simulink model "3_ZSM"  (R2016a)
settings: Solver=ode1  StartTime=0.0  StopTime=t_sim  FixedStep=0.001  RelTol=1e-3
values from neighbouring files (symbols this model uses):
  A = 1.5    [3_ZSM_Parameters.m]
  C = 1.3    [2_ESM_Parameters.m]    (also in 3_ZSM_Parameters.m)
  c_h_l = 0.5 * c_h    (= 71619.7243914)    [3_ZSM_Parameters.m]
  c_h_r = 0.5 * c_h    (= 71619.7243914)    [3_ZSM_Parameters.m]
  c_v_l = 0.5 * c_v    (= 39054.886799)    [3_ZSM_Parameters.m]
  c_v_r = 0.5 * c_v    (= 39054.886799)    [3_ZSM_Parameters.m]
  c_w = 0.4    [3_ZSM_Parameters.m]
  dynamicload_mode = i-1    [3_ZSM_Parameters.m]
  E = 0.85    [2_ESM_Parameters.m]    (also in 3_ZSM_Parameters.m)
  f_x_init = 0.5*A*c_w*rho*v_init^2    (= 24.980004)    [3_ZSM_Parameters.m]
  fz1 = fz(:,1)    [3_ZSM_Parameters.m]
  g = 9.81    [3_ZSM_Parameters.m]
  h_s = 0.5    [3_ZSM_Parameters.m]
  L = 2.71    [2_ESM_Parameters.m]    (also in 3_ZSM_Parameters.m)
  l_h = m_v * L / m    (= 1.35481930924)    [2_ESM_Parameters.m]    (also in 3_ZSM_Parameters.m)
  l_v = m_h * L / m    (= 1.35518069076)    [2_ESM_Parameters.m]    (also in 3_ZSM_Parameters.m)
  m = m_v + m_h    (= 1499.8)    [2_ESM_Parameters.m]    (also in 3_ZSM_Parameters.m)
  m_hl = m * l_v / L * SP_yl    (= 375)    [3_ZSM_Parameters.m]
  m_hr = m * l_v / L * SP_yr    (= 375)    [3_ZSM_Parameters.m]
  m_vl = m * l_h / L * SP_yl    (= 374.9)    [3_ZSM_Parameters.m]
  m_vr = m * l_h / L * SP_yr    (= 374.9)    [3_ZSM_Parameters.m]
  mu = 0.9    [2_ESM_Parameters.m]    (also in 3_ZSM_Parameters.m)
  rho = 1.2    [3_ZSM_Parameters.m]
  s_h = 1.57    [3_ZSM_Parameters.m]
  s_v = 1.54    [3_ZSM_Parameters.m]
  SP_yl = 0.5    [3_ZSM_Parameters.m]
  SP_yr = 1 - SP_yl    (= 0.5)    [3_ZSM_Parameters.m]
  v = setting(i,3)    [2_ESM_Parameters.m]
  v_init = 8.33    [3_ZSM_Parameters.m]
undefined symbols (not defined in the file or in its folder): Delta, fz
undefined symbols (not defined in the file): Lenkwinkel, Radlenkwinkel, T_z
libraries: simulink x2
(part 2 of 2)

== system 3_ZSM/Even Two-Track Model/Determine wheel movement/Calculate slip angle rear left ==
  Vehicle Bus : Inport
  Calculated Inputs : Inport  Port=2
  Bus Selector : BusSelector  OutputSignals=Steering_Bus.Delta_h_l
  Bus Selector1 : BusSelector  OutputSignals=v_beta_sin,psi_p_l_rear
  Bus Selector2 : BusSelector  OutputSignals=v_beta_cos,psi_p_tw_rear
  Divide : Product  Inputs=*/
  Sum : Sum  Inputs=+-  SaturateOnIntegerOverflow=on
  Sum1 : Sum  Inputs=+-  SaturateOnIntegerOverflow=on
  Sum2 : Sum  Inputs=+-  SaturateOnIntegerOverflow=on
  Trigonometric Function : Trigonometry  Operator=atan
  alpha_rear_left [rad] : Outport
  wires:
  Bus Selector2/1 -> Sum1/1  "<v_beta_cos>"
  Calculated Inputs/1 -> Bus Selector1/1, Bus Selector2/1
  Bus Selector2/2 -> Sum1/2  "<psi_p_tw_rear>"
  Sum1/1 -> Divide/2
  Bus Selector1/2 -> Sum2/2  "<psi_p_l_rear>"
  Bus Selector1/1 -> Sum2/1  "<v_beta_sin>"
  Sum2/1 -> Divide/1
  Trigonometric Function/1 -> Sum/2
  Divide/1 -> Trigonometric Function/1
  Vehicle Bus/1 -> Bus Selector/1
  Sum/1 -> alpha_rear_left [rad]/1
  Bus Selector/1 -> Sum/1  "<Delta_h_l>"

== system 3_ZSM/Even Two-Track Model/Determine wheel movement/Calculate slip angle rear right ==
  Vehicle Bus : Inport
  Calculated Inputs : Inport  Port=2
  Bus Selector : BusSelector  OutputSignals=Steering_Bus.Delta_h_r
  Bus Selector1 : BusSelector  OutputSignals=v_beta_sin,psi_p_l_rear
  Bus Selector2 : BusSelector  OutputSignals=v_beta_cos,psi_p_tw_rear
  Divide : Product  Inputs=*/
  Sum : Sum  Inputs=+-  SaturateOnIntegerOverflow=on
  Sum1 : Sum  SaturateOnIntegerOverflow=on
  Sum2 : Sum  Inputs=+-  SaturateOnIntegerOverflow=on
  Trigonometric Function : Trigonometry  Operator=atan
  alpha_rear_right [rad] : Outport
  wires:
  Bus Selector2/1 -> Sum1/1  "<v_beta_cos>"
  Calculated Inputs/1 -> Bus Selector1/1, Bus Selector2/1
  Bus Selector2/2 -> Sum1/2  "<psi_p_tw_rear>"
  Sum1/1 -> Divide/2
  Bus Selector1/2 -> Sum2/2  "<psi_p_l_rear>"
  Bus Selector1/1 -> Sum2/1  "<v_beta_sin>"
  Sum2/1 -> Divide/1
  Trigonometric Function/1 -> Sum/2
  Divide/1 -> Trigonometric Function/1
  Vehicle Bus/1 -> Bus Selector/1
  Sum/1 -> alpha_rear_right [rad]/1
  Bus Selector/1 -> Sum/1  "<Delta_h_r>"

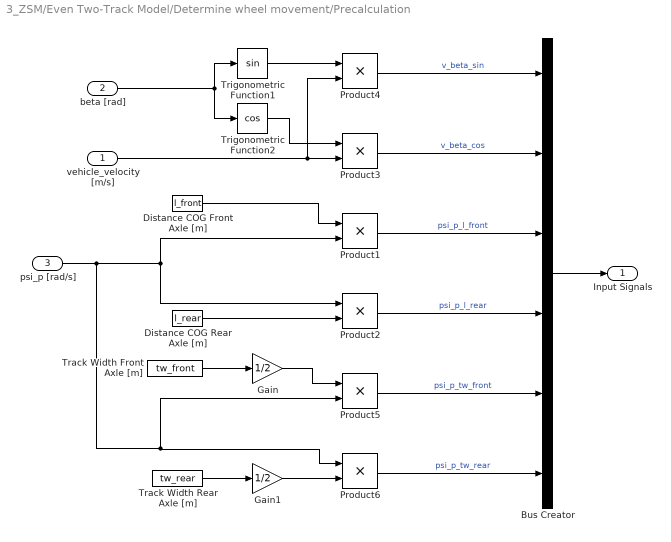
== system 3_ZSM/Even Two-Track Model/Determine wheel movement/Precalculation ==
  vehicle_velocity [m/s] : Inport
  beta [rad] : Inport  Port=2
  psi_p [rad/s] : Inport  Port=3
  Bus Creator : BusCreator  Inputs=6
  Distance COG Front Axle [m] : Constant  Value=l_front
  Distance COG Rear Axle [m] : Constant  Value=l_rear
  Gain : Gain  Gain=1/2
  Gain1 : Gain  Gain=1/2
  Product{1..6} (6 alike) : Product  SaturateOnIntegerOverflow=on  OutDataTypeStr=Inherit: Same as first input
  Track Width Front Axle [m] : Constant  Value=tw_front
  Track Width Rear Axle [m] : Constant  Value=tw_rear
  Trigonometric Function1 : Trigonometry
  Trigonometric Function2 : Trigonometry  Operator=cos
  Input Signals : Outport
  wires:
  Product1/1 -> Bus Creator/3  "psi_p_l_front"
  Gain1/1 -> Product6/2
  Product4/1 -> Bus Creator/1  "v_beta_sin"
  Gain/1 -> Product5/1
  Track Width Front Axle [m]/1 -> Gain/1
  Product5/1 -> Bus Creator/5  "psi_p_tw_front"
  Track Width Rear Axle [m]/1 -> Gain1/1
  Trigonometric Function1/1 -> Product4/1
  psi_p [rad/s]/1 -> Product1/2, Product2/1, Product5/2, Product6/1
  Trigonometric Function2/1 -> Product3/1
  vehicle_velocity [m/s]/1 -> Product3/2, Product4/2
  Product2/1 -> Bus Creator/4  "psi_p_l_rear"
  Product6/1 -> Bus Creator/6  "psi_p_tw_rear"
  Product3/1 -> Bus Creator/2  "v_beta_cos"
  beta [rad]/1 -> Trigonometric Function1/1, Trigonometric Function2/1
  Bus Creator/1 -> Input Signals/1
  Distance COG Front Axle [m]/1 -> Product1/1
  Distance COG Rear Axle [m]/1 -> Product2/2

== system 3_ZSM/Tire/Tire front left/Kammscher Kreis ==
  F_z_FL [N] : Inport
  F_x_FL [N] : Inport  Port=2
  1-D Lookup Table : Lookup_n-D  NumberOfTableDimensions=1  BreakpointsForDimension1=fz1  Table=fz  InternalRulePriority=Speed  RndMeth=Simplest  InputSameDT=on
  Add : Sum  Inputs=+-
  Math Function : Math  Operator=square  SaturateOnIntegerOverflow=on
  Math Function1 : Math  Operator=square  SaturateOnIntegerOverflow=on
  Sqrt : Sqrt  SaturateOnIntegerOverflow=on
  Sqrt1 : Sqrt  SaturateOnIntegerOverflow=on
  F_y_v_l_max [N] : Outport
  F_v_l_max [N] : Outport  Port=2
  wires:
  F_z_FL [N]/1 -> 1-D Lookup Table/1
  Math Function/1 -> Add/2
  Math Function1/1 -> Sqrt1/1, Add/1
  1-D Lookup Table/1 -> Math Function1/1  "F_x_max"
  F_x_FL [N]/1 -> Math Function/1
  Add/1 -> Sqrt/1  "F_y_max"
  Sqrt/1 -> F_y_v_l_max [N]/1
  Sqrt1/1 -> F_v_l_max [N]/1

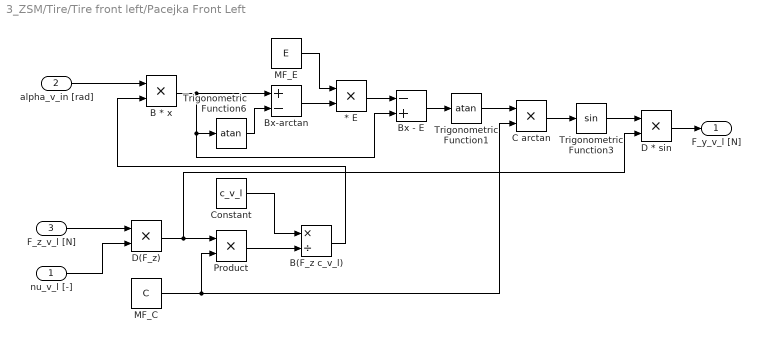
== system 3_ZSM/Tire/Tire front left/Pacejka Front Left ==
  nu_v_l [-] : Inport
  alpha_v_in [rad] : Inport  Port=2
  F_z_v_l [N] : Inport  Port=3
  * E : Product
  B * x : Product
  B(F_z c_v_l) : Product  Inputs=*/
  Bx - E : Sum  Inputs=-+
  Bx-arctan : Sum  Inputs=+-
  C arctan : Product
  Constant : Constant  Value=c_v_l
  D * sin : Product
  D(F_z) : Product
  MF_C : Constant  Value=C
  MF_E : Constant  Value=E
  Product : Product
  Trigonometric Function1 : Trigonometry  Operator=atan
  Trigonometric Function3 : Trigonometry
  Trigonometric Function6 : Trigonometry  Operator=atan
  F_y_v_l [N] : Outport
  wires:
  D * sin/1 -> F_y_v_l [N]/1
  Trigonometric Function6/1 -> Bx-arctan/2
  C arctan/1 -> Trigonometric Function3/1
  B * x/1 -> Bx-arctan/1, Bx - E/2, Trigonometric Function6/1
  Bx - E/1 -> Trigonometric Function1/1
  Bx-arctan/1 -> * E/2
  MF_E/1 -> * E/1
  * E/1 -> Bx - E/1
  F_z_v_l [N]/1 -> D(F_z)/1
  nu_v_l [-]/1 -> D(F_z)/2
  Product/1 -> B(F_z c_v_l)/2
  Constant/1 -> B(F_z c_v_l)/1
  D(F_z)/1 -> D * sin/2, Product/1
  MF_C/1 -> C arctan/2, Product/2
  B(F_z c_v_l)/1 -> B * x/2
  Trigonometric Function1/1 -> C arctan/1
  Trigonometric Function3/1 -> D * sin/1
  alpha_v_in [rad]/1 -> B * x/1

== system 3_ZSM/Tire/Tire front right/Kammscher Kreis ==
  F_z_v_r [N] : Inport
  F_x_v_r [N] : Inport  Port=2
  1-D Lookup Table : Lookup_n-D  NumberOfTableDimensions=1  BreakpointsForDimension1=fz1  Table=fz  InternalRulePriority=Speed  RndMeth=Simplest  InputSameDT=on
  Add : Sum  Inputs=+-
  Math Function : Math  Operator=square  SaturateOnIntegerOverflow=on
  Math Function1 : Math  Operator=square  SaturateOnIntegerOverflow=on
  Sqrt : Sqrt  SaturateOnIntegerOverflow=on
  Sqrt1 : Sqrt  SaturateOnIntegerOverflow=on
  F_y_v_r_max [N] : Outport
  F_v_r_max [N] : Outport  Port=2
  wires:
  F_z_v_r [N]/1 -> 1-D Lookup Table/1
  Math Function/1 -> Add/2
  1-D Lookup Table/1 -> Math Function1/1  "F_x_max"
  F_x_v_r [N]/1 -> Math Function/1
  Add/1 -> Sqrt/1  "F_y_max"
  Sqrt/1 -> F_y_v_r_max [N]/1
  Math Function1/1 -> Sqrt1/1, Add/1
  Sqrt1/1 -> F_v_r_max [N]/1

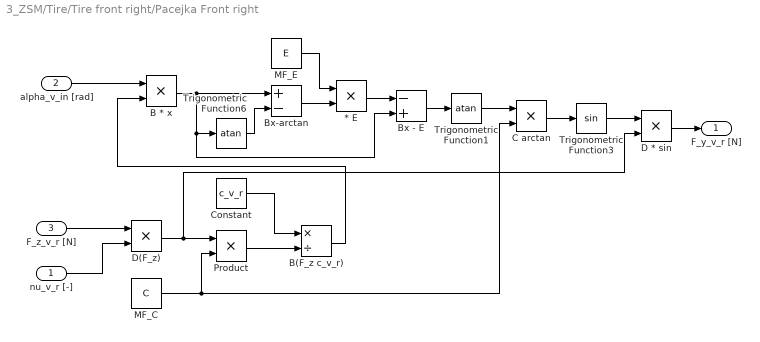
== system 3_ZSM/Tire/Tire front right/Pacejka Front right ==
  nu_v_r [-] : Inport
  alpha_v_in [rad] : Inport  Port=2
  F_z_v_r [N] : Inport  Port=3
  * E : Product
  B * x : Product
  B(F_z c_v_r) : Product  Inputs=*/
  Bx - E : Sum  Inputs=-+
  Bx-arctan : Sum  Inputs=+-
  C arctan : Product
  Constant : Constant  Value=c_v_r
  D * sin : Product
  D(F_z) : Product
  MF_C : Constant  Value=C
  MF_E : Constant  Value=E
  Product : Product
  Trigonometric Function1 : Trigonometry  Operator=atan
  Trigonometric Function3 : Trigonometry
  Trigonometric Function6 : Trigonometry  Operator=atan
  F_y_v_r [N] : Outport
  wires:
  D * sin/1 -> F_y_v_r [N]/1
  Trigonometric Function6/1 -> Bx-arctan/2
  C arctan/1 -> Trigonometric Function3/1
  B * x/1 -> Bx-arctan/1, Bx - E/2, Trigonometric Function6/1
  Bx - E/1 -> Trigonometric Function1/1
  Bx-arctan/1 -> * E/2
  MF_E/1 -> * E/1
  * E/1 -> Bx - E/1
  F_z_v_r [N]/1 -> D(F_z)/1
  nu_v_r [-]/1 -> D(F_z)/2
  Product/1 -> B(F_z c_v_r)/2
  Constant/1 -> B(F_z c_v_r)/1
  D(F_z)/1 -> D * sin/2, Product/1
  MF_C/1 -> C arctan/2, Product/2
  B(F_z c_v_r)/1 -> B * x/2
  Trigonometric Function1/1 -> C arctan/1
  Trigonometric Function3/1 -> D * sin/1
  alpha_v_in [rad]/1 -> B * x/1

== system 3_ZSM/Tire/Tire rear left/Kammscher Kreis ==
  F_z_h_l [N] : Inport
  F_x_h_l [N] : Inport  Port=2
  1-D Lookup Table : Lookup_n-D  NumberOfTableDimensions=1  BreakpointsForDimension1=fz1  Table=fz  InternalRulePriority=Speed  RndMeth=Simplest  InputSameDT=on
  Add : Sum  Inputs=+-
  Math Function : Math  Operator=square  SaturateOnIntegerOverflow=on
  Math Function1 : Math  Operator=square  SaturateOnIntegerOverflow=on
  Sqrt : Sqrt  SaturateOnIntegerOverflow=on
  Sqrt1 : Sqrt  SaturateOnIntegerOverflow=on
  F_y_h_l_max [N] : Outport
  F_h_l_max [N] : Outport  Port=2
  wires:
  F_z_h_l [N]/1 -> 1-D Lookup Table/1
  Math Function/1 -> Add/2
  1-D Lookup Table/1 -> Math Function1/1  "F_x_max"
  F_x_h_l [N]/1 -> Math Function/1
  Add/1 -> Sqrt/1  "F_y_max"
  Sqrt/1 -> F_y_h_l_max [N]/1
  Math Function1/1 -> Sqrt1/1, Add/1
  Sqrt1/1 -> F_h_l_max [N]/1

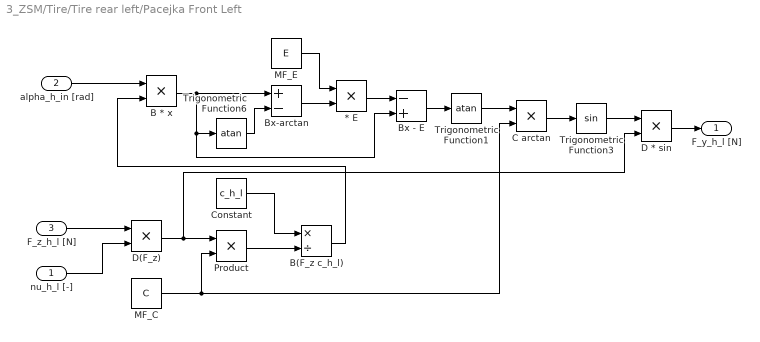
== system 3_ZSM/Tire/Tire rear left/Pacejka Front Left ==
  nu_h_l [-] : Inport
  alpha_h_in [rad] : Inport  Port=2
  F_z_h_l [N] : Inport  Port=3
  * E : Product
  B * x : Product
  B(F_z c_h_l) : Product  Inputs=*/
  Bx - E : Sum  Inputs=-+
  Bx-arctan : Sum  Inputs=+-
  C arctan : Product
  Constant : Constant  Value=c_h_l
  D * sin : Product
  D(F_z) : Product
  MF_C : Constant  Value=C
  MF_E : Constant  Value=E
  Product : Product
  Trigonometric Function1 : Trigonometry  Operator=atan
  Trigonometric Function3 : Trigonometry
  Trigonometric Function6 : Trigonometry  Operator=atan
  F_y_h_l [N] : Outport
  wires:
  D * sin/1 -> F_y_h_l [N]/1
  Trigonometric Function6/1 -> Bx-arctan/2
  C arctan/1 -> Trigonometric Function3/1
  B * x/1 -> Bx-arctan/1, Bx - E/2, Trigonometric Function6/1
  Bx - E/1 -> Trigonometric Function1/1
  Bx-arctan/1 -> * E/2
  MF_E/1 -> * E/1
  * E/1 -> Bx - E/1
  F_z_h_l [N]/1 -> D(F_z)/1
  nu_h_l [-]/1 -> D(F_z)/2
  Product/1 -> B(F_z c_h_l)/2
  Constant/1 -> B(F_z c_h_l)/1
  D(F_z)/1 -> D * sin/2, Product/1
  MF_C/1 -> C arctan/2, Product/2
  B(F_z c_h_l)/1 -> B * x/2
  Trigonometric Function1/1 -> C arctan/1
  Trigonometric Function3/1 -> D * sin/1
  alpha_h_in [rad]/1 -> B * x/1

== system 3_ZSM/Tire/Tire rear right/Kammscher Kreis ==
  F_z_h_r [N] : Inport
  F_x_h_r [N] : Inport  Port=2
  1-D Lookup Table : Lookup_n-D  NumberOfTableDimensions=1  BreakpointsForDimension1=fz1  Table=fz  InternalRulePriority=Speed  RndMeth=Simplest  InputSameDT=on
  Add : Sum  Inputs=+-
  Math Function : Math  Operator=square  SaturateOnIntegerOverflow=on
  Math Function1 : Math  Operator=square  SaturateOnIntegerOverflow=on
  Sqrt : Sqrt  SaturateOnIntegerOverflow=on
  Sqrt1 : Sqrt  SaturateOnIntegerOverflow=on
  F_y_h_r_max [N] : Outport
  F_h_r_max [N] : Outport  Port=2
  wires:
  F_z_h_r [N]/1 -> 1-D Lookup Table/1
  Math Function/1 -> Add/2
  1-D Lookup Table/1 -> Math Function1/1  "F_x_max"
  F_x_h_r [N]/1 -> Math Function/1
  Add/1 -> Sqrt/1  "F_y_max"
  Sqrt/1 -> F_y_h_r_max [N]/1
  Math Function1/1 -> Sqrt1/1, Add/1
  Sqrt1/1 -> F_h_r_max [N]/1

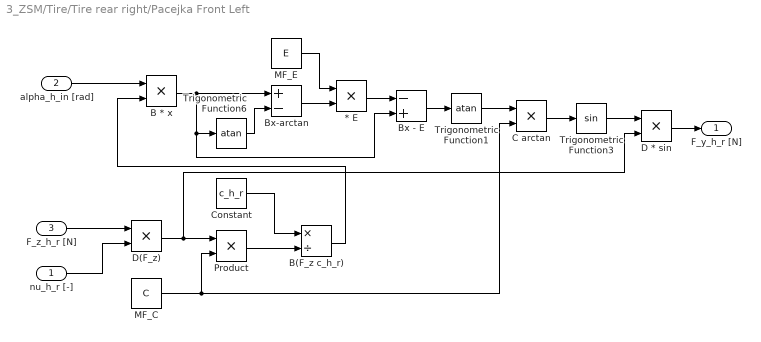
== system 3_ZSM/Tire/Tire rear right/Pacejka Front Left ==
  nu_h_r [-] : Inport
  alpha_h_in [rad] : Inport  Port=2
  F_z_h_r [N] : Inport  Port=3
  * E : Product
  B * x : Product
  B(F_z c_h_r) : Product  Inputs=*/
  Bx - E : Sum  Inputs=-+
  Bx-arctan : Sum  Inputs=+-
  C arctan : Product
  Constant : Constant  Value=c_h_r
  D * sin : Product
  D(F_z) : Product
  MF_C : Constant  Value=C
  MF_E : Constant  Value=E
  Product : Product
  Trigonometric Function1 : Trigonometry  Operator=atan
  Trigonometric Function3 : Trigonometry
  Trigonometric Function6 : Trigonometry  Operator=atan
  F_y_h_r [N] : Outport
  wires:
  D * sin/1 -> F_y_h_r [N]/1
  Trigonometric Function6/1 -> Bx-arctan/2
  C arctan/1 -> Trigonometric Function3/1
  B * x/1 -> Bx-arctan/1, Bx - E/2, Trigonometric Function6/1
  Bx - E/1 -> Trigonometric Function1/1
  Bx-arctan/1 -> * E/2
  MF_E/1 -> * E/1
  * E/1 -> Bx - E/1
  F_z_h_r [N]/1 -> D(F_z)/1
  nu_h_r [-]/1 -> D(F_z)/2
  Product/1 -> B(F_z c_h_r)/2
  Constant/1 -> B(F_z c_h_r)/1
  D(F_z)/1 -> D * sin/2, Product/1
  MF_C/1 -> C arctan/2, Product/2
  B(F_z c_h_r)/1 -> B * x/2
  Trigonometric Function1/1 -> C arctan/1
  Trigonometric Function3/1 -> D * sin/1
  alpha_h_in [rad]/1 -> B * x/1
